simulink model "LinearizedQuadModel"  (R2015b)
settings: Solver=ode45  StartTime=0.0  StopTime=400  RelTol=1e-3
values from neighbouring files (symbols this model uses):
  b_ = 3.13E-5    (= 3.13e-05)    [LinearizedQuad.m]
  Iyy = 6.228E-3    (= 0.006228)    [LinearizedQuad.m]
  Klqr_i = lqr(A_aug,B_aug, Q2, R)    [LinearizedQuad.m]
  Klqr_i_2 = lqr(A_aug2,B_aug2, Q_2i, R_2)    [LinearizedQuad.m]
  Klqr_x = lqr(Ax, Bx, Qx, Rx)    [LinearizedQuad.m]
  l = 0.232    [LinearizedQuad.m]
  m = 0.53    [LinearizedQuad.m]
undefined symbols (not defined in the file or in its folder): deg, rad, s
libraries: aerolibconvert2 x7, simulink x1
settings Model: Creator=aa13417  LastModifiedBy=Salua
settings DataIOCC: SaveFormat=Array
settings DebuggingCC: UnderspecifiedInitializationDetection=Classic  MergeDetectMultiDrivingBlocksExec=none  SolverPrmCheckMsg=warning  StateNameClashWarn=warning
settings HardwareCC: ProdBitPerPointer=32  ProdLargestAtomicFloat=None  ProdIntDivRoundTo=Undefined  ProdEndianess=Unspecified  ProdWordSize=32  ProdHWDeviceType=32-bit Generic
settings GRTTargetCC: GeneratePreprocessorConditionals=Disable all
settings ConfigComp: CovModelRefEnable=Off

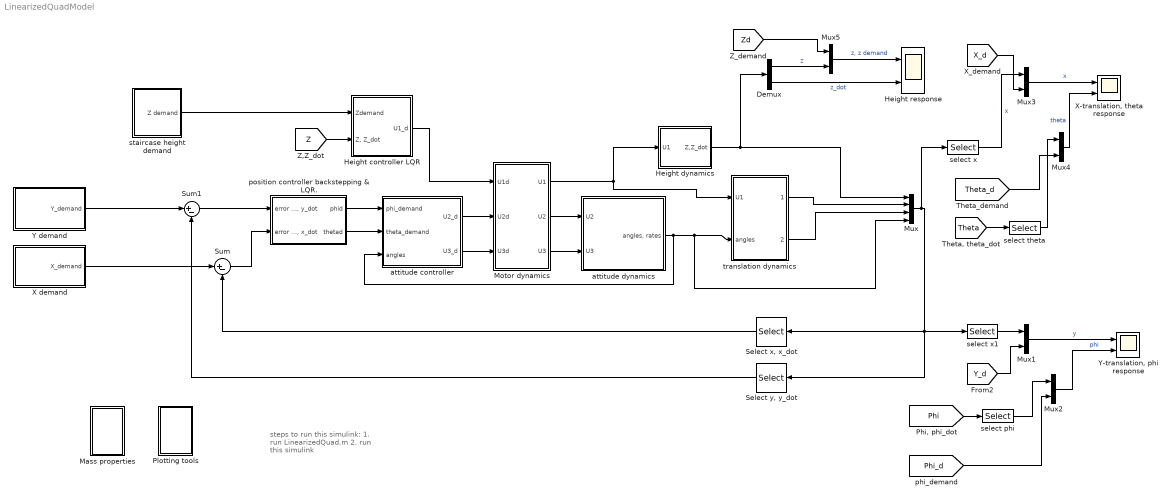
== system LinearizedQuadModel ==
  note: steps to run this simulink:
      | 1. run LinearizedQuad.m
      | 2. run this simulink
  Demux : Demux  Outputs=2
  Height controller LQR : Subsystem
  Height dynamics : Subsystem
  Height response : Scope  NumInputPorts=2
  Mass properties : Subsystem
  Motor dynamics : Subsystem
  Mux : Mux
  Mux{1..5} (5 alike) : Mux  Inputs=2
  Plotting tools : Subsystem
  "Select x, x_dot" : Selector  InputPortWidth=10  IndexOptions=Index vector (dialog)  Indices=[3, 4]  OutputSizes=1
  "Select y, y_dot" : Selector  InputPortWidth=10  IndexOptions=Index vector (dialog)  Indices=[5, 6]  OutputSizes=1
  Sum : Sum  Inputs=|+-
  Sum1 : Sum  Inputs=|+-
  "X demand " : Subsystem
  "X-translation, theta response" : Scope  NumInputPorts=2
  "Y demand " : Subsystem
  "Y-translation, phi response" : Scope  NumInputPorts=2
  attitude controller : Subsystem
  attitude dynamics : Subsystem
  position controller backstepping & LQR. : Subsystem
  select phi : Selector  InputPortWidth=2  IndexOptions=Index vector (dialog)  Indices=1  OutputSizes=1
  select theta : Selector  InputPortWidth=2  IndexOptions=Index vector (dialog)  Indices=1  OutputSizes=1
  select x : Selector  InputPortWidth=10  IndexOptions=Index vector (dialog)  Indices=3  OutputSizes=1
  select x1 : Selector  InputPortWidth=10  IndexOptions=Index vector (dialog)  Indices=5  OutputSizes=1
  staircase height demand : Subsystem
  translation dynamics : Subsystem
  wires:
  Height dynamics/1(Z,Z_dot) -> Mux/1, Demux/1
  attitude dynamics/1("angles, rates") -> attitude controller/3(angles), Mux/4, translation dynamics/2(angles)
  translation dynamics/1("X, X_dot") -> Mux/2
  Mux/1 -> select x/1, select x1/1, "Select x, x_dot"/1, "Select y, y_dot"/1
  "Select x, x_dot"/1 -> Sum/2
  Height controller LQR/1(U1_d) -> Motor dynamics/1(U1d)
  attitude controller/2(U3_d) -> Motor dynamics/3(U3d)
  Motor dynamics/1(U1) -> translation dynamics/1(U1), Height dynamics/1(U1)
  Demux/2 -> Height response/2  "z_dot"
  [Z] -> Height controller LQR/2("Z, Z_dot")
  Motor dynamics/3(U3) -> attitude dynamics/2(U3)
  translation dynamics/2("Y, Y_dot") -> Mux/3
  "Select y, y_dot"/1 -> Sum1/2
  attitude controller/1(U2_d) -> Motor dynamics/2(U2d)
  Motor dynamics/2(U2) -> attitude dynamics/1("U2 ")
  staircase height demand/1(Z demand) -> Height controller LQR/1(Zdemand)
  select x/1 -> Mux3/1  "x"
  [X_d] -> Mux3/2
  Mux3/1 -> "X-translation, theta response"/1  "x"
  [Theta_d] -> Mux4/2
  Mux4/1 -> "X-translation, theta response"/2  "theta"
  [Theta] -> select theta/1
  select theta/1 -> Mux4/1
  position controller backstepping & LQR./2(thetad) -> attitude controller/2(theta_demand)
  position controller backstepping & LQR./1(phid) -> attitude controller/1(phi_demand)
  select x1/1 -> Mux1/1
  [Y_d] -> Mux1/2
  Mux1/1 -> "Y-translation, phi response"/1  "y"
  Mux2/1 -> "Y-translation, phi response"/2  "phi"
  [Phi] -> select phi/1
  select phi/1 -> Mux2/1
  [Phi_d] -> Mux2/2
  [Zd] -> Mux5/1
  Demux/1 -> Mux5/2  "z"
  Mux5/1 -> Height response/1  "z, z demand"
  "Y demand "/1(Y_demand) -> Sum1/1
  "X demand "/1(X_demand) -> Sum/1
  Sum1/1 -> position controller backstepping & LQR./1("error y, y_dot")
  Sum/1 -> position controller backstepping & LQR./2("error x, x_dot")

== system LinearizedQuadModel/Height controller LQR ==
  Zdemand : Inport
  "Z, Z_dot" : Inport  Port=2
  LQR control : Subsystem
  U1_d : Outport
  wires:
  Zdemand/1 -> LQR control/1(Zd)
  LQR control/1(U1d) -> U1_d/1
  "Z, Z_dot"/1 -> LQR control/2(states)

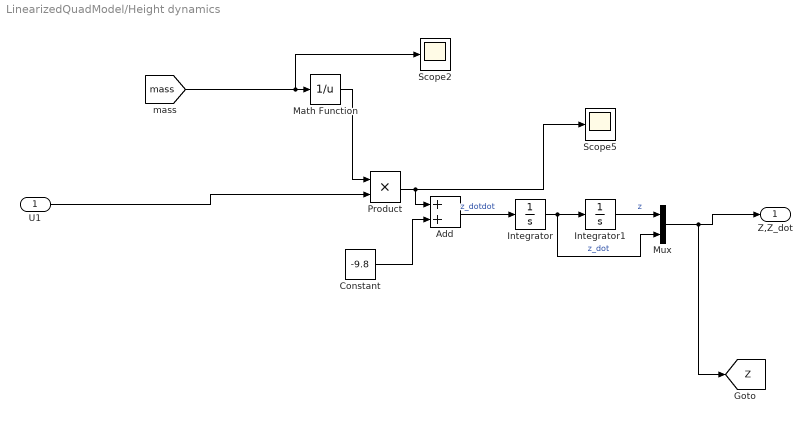
== system LinearizedQuadModel/Height dynamics ==
  U1 : Inport
  Add : Sum
  Constant : Constant  Value=-9.8
  Integrator : Integrator
  Integrator1 : Integrator
  Math Function : Math  Operator=reciprocal  SaturateOnIntegerOverflow=on
  Mux : Mux  Inputs=2
  Product : Product
  Scope2 : Scope
  Scope5 : Scope
  Z,Z_dot : Outport
  tag scope: Z=global
  wires:
  Integrator/1 -> Mux/2, Integrator1/1  "z_dot"
  Product/1 -> Scope5/1, Add/1
  [mass] -> Scope2/1, Math Function/1
  Math Function/1 -> Product/1
  Integrator1/1 -> Mux/1  "z"
  Mux/1 -> [Z], Z,Z_dot/1
  Add/1 -> Integrator/1  "z_dotdot"
  Constant/1 -> Add/2
  U1/1 -> Product/2

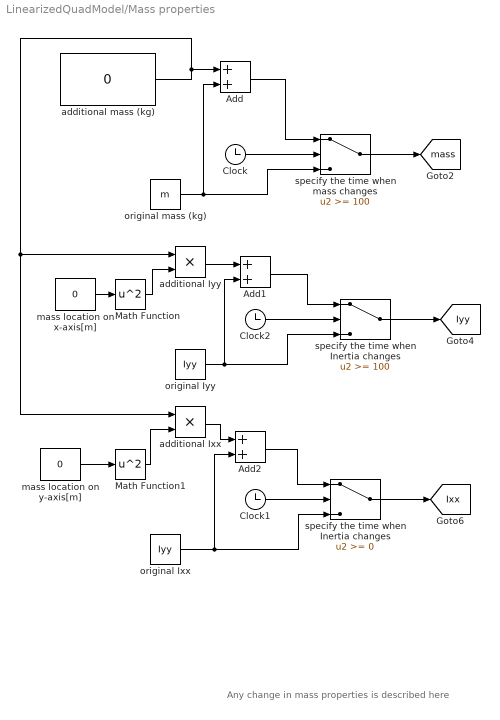
== system LinearizedQuadModel/Mass properties ==
  note: Any change in mass properties is described here
  Add : Sum
  Add1 : Sum
  Add2 : Sum
  Clock : Clock
  Clock1 : Clock
  Clock2 : Clock
  Math Function : Math  Operator=square  SaturateOnIntegerOverflow=on
  Math Function1 : Math  Operator=square  SaturateOnIntegerOverflow=on
  additional Ixx : Product  Inputs=**
  additional Iyy : Product  Inputs=**
  additional mass (kg) : Constant  Value=0
  mass location on x-axis[m] : Constant  Value=0
  mass location on y-axis[m] : Constant  Value=0
  original Ixx : Constant  Value=Iyy
  original Iyy : Constant  Value=Iyy
  original mass (kg) : Constant  Value=m
  specify the time when Inertia changes : Switch  Threshold=100
  "specify the time when Inertia changes  " : Switch
  specify the time when mass changes : Switch  Threshold=100
  tag scope: Ixx=global, Iyy=global, mass=global
  wires:
  Add/1 -> specify the time when mass changes/1
  specify the time when mass changes/1 -> [mass]
  original mass (kg)/1 -> specify the time when mass changes/3, Add/2
  Clock/1 -> specify the time when mass changes/2
  Add1/1 -> specify the time when Inertia changes/1
  specify the time when Inertia changes/1 -> [Iyy]
  original Iyy/1 -> Add1/2, specify the time when Inertia changes/3
  Clock2/1 -> specify the time when Inertia changes/2
  additional mass (kg)/1 -> additional Iyy/1, additional Ixx/1, Add/1
  mass location on x-axis[m]/1 -> Math Function/1
  additional Iyy/1 -> Add1/1
  "specify the time when Inertia changes  "/1 -> [Ixx]
  Clock1/1 -> "specify the time when Inertia changes  "/2
  original Ixx/1 -> Add2/2, "specify the time when Inertia changes  "/3
  Add2/1 -> "specify the time when Inertia changes  "/1
  mass location on y-axis[m]/1 -> Math Function1/1
  additional Ixx/1 -> Add2/1
  Math Function/1 -> additional Iyy/2
  Math Function1/1 -> additional Ixx/2

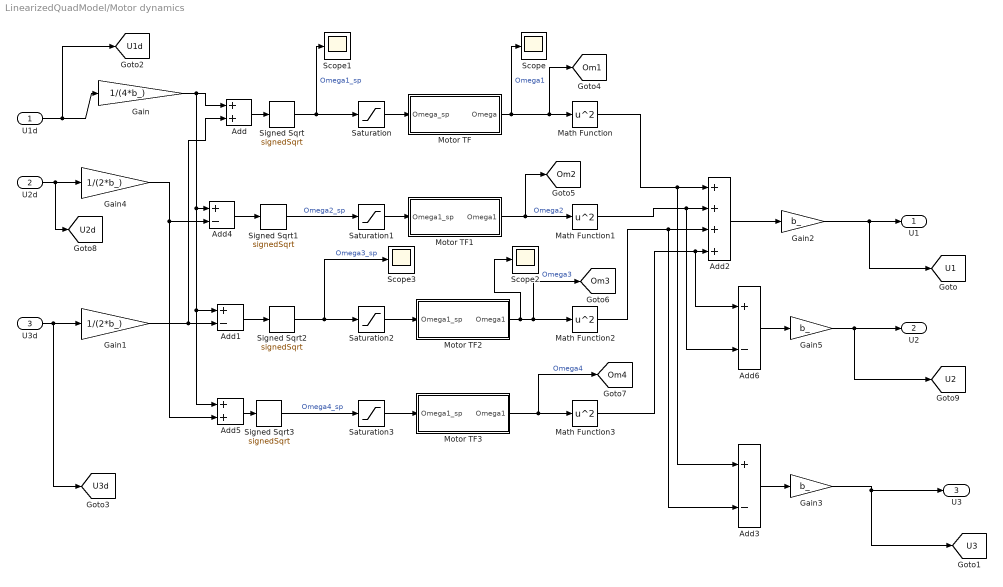
== system LinearizedQuadModel/Motor dynamics ==
  U1d : Inport
  U2d : Inport  Port=2
  U3d : Inport  Port=3
  Add : Sum
  Add{1,3..4,6} (4 alike) : Sum  Inputs=+-
  Add2 : Sum  Inputs=++++
  Add5 : Sum
  Gain : Gain  Gain=1/(4*b_)
  Gain1 : Gain  Gain=1/(2*b_)
  Gain2 : Gain  Gain=b_
  Gain3 : Gain  Gain=b_
  Gain4 : Gain  Gain=1/(2*b_)
  Gain5 : Gain  Gain=b_
  Math Function{,1..3} (4 alike) : Math  Operator=square  SaturateOnIntegerOverflow=on
  Motor TF : Subsystem
  Motor TF1 : Subsystem
  Motor TF2 : Subsystem
  Motor TF3 : Subsystem
  Saturation{,1..3} (4 alike) : Saturate  UpperLimit=341  LowerLimit=24
  Scope{,1..3} (4 alike) : Scope
  Signed Sqrt{,1..3} (4 alike) : Sqrt  Operator=signedSqrt  OutputSignalType=real  SaturateOnIntegerOverflow=on
  U1 : Outport
  U2 : Outport  Port=2
  U3 : Outport  Port=3
  tag scope: Om1=global, Om2=global, Om3=global, Om4=global, U1=global, U1d=global, U2=global, U2d=global, U3=global, U3d=global
  wires:
  U3d/1 -> [U3d], Gain1/1
  Motor TF/1(Omega) -> Scope/1, [Om1], Math Function/1  "Omega1"
  Saturation/1 -> Motor TF/1(Omega_sp)
  Gain/1 -> Add5/1, Add1/1, Add4/1, Add/1
  U1d/1 -> [U1d], Gain/1
  Add/1 -> Signed Sqrt/1
  Math Function/1 -> Add2/1, Add3/1
  Signed Sqrt/1 -> Scope1/1, Saturation/1  "Omega1_sp"
  Gain1/1 -> Add/2, Add1/2
  Signed Sqrt1/1 -> Saturation1/1  "Omega2_sp"
  Saturation1/1 -> Motor TF1/1(Omega1_sp)
  Add1/1 -> Signed Sqrt2/1
  Signed Sqrt2/1 -> Scope3/1, Saturation2/1  "Omega3_sp"
  Saturation2/1 -> Motor TF2/1(Omega1_sp)
  Motor TF2/1(Omega1) -> Scope2/1, [Om3], Math Function2/1  "Omega3"
  Signed Sqrt3/1 -> Saturation3/1  "Omega4_sp"
  Saturation3/1 -> Motor TF3/1(Omega1_sp)
  Motor TF3/1(Omega1) -> [Om4], Math Function3/1  "Omega4"
  Math Function3/1 -> Add6/1, Add2/4
  Math Function2/1 -> Add3/2, Add2/3
  Math Function1/1 -> Add2/2, Add6/2
  Add2/1 -> Gain2/1
  Gain2/1 -> [U1], U1/1
  Add3/1 -> Gain3/1
  Gain3/1 -> U3/1, [U3]
  Motor TF1/1(Omega1) -> [Om2], Math Function1/1  "Omega2"
  U2d/1 -> Gain4/1, [U2d]
  Gain4/1 -> Add5/2, Add4/2
  Add4/1 -> Signed Sqrt1/1
  Add5/1 -> Signed Sqrt3/1
  Add6/1 -> Gain5/1
  Gain5/1 -> [U2], U2/1

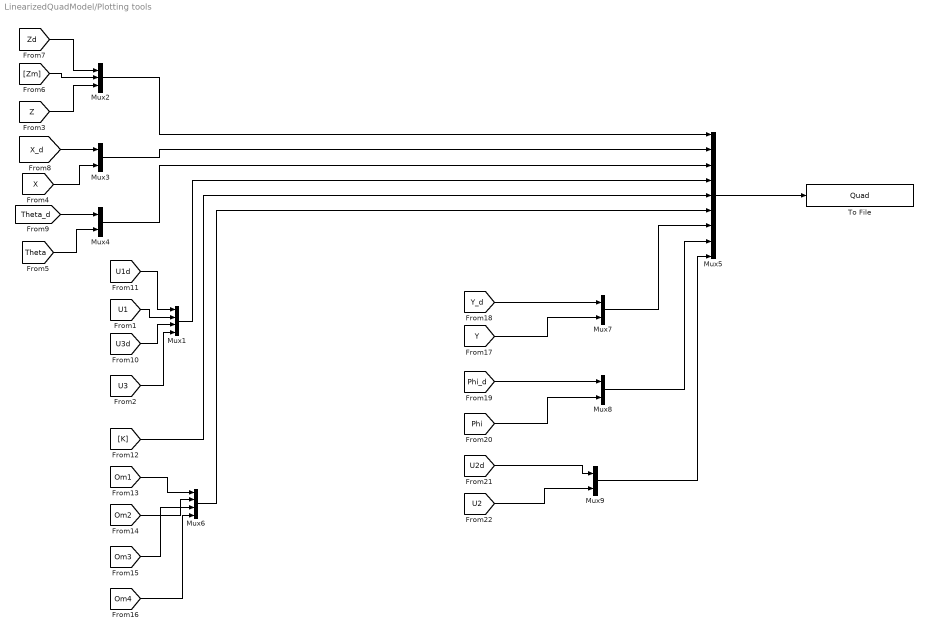
== system LinearizedQuadModel/Plotting tools ==
  Mux1 : Mux
  Mux2 : Mux  Inputs=3
  Mux{3..4,7..9} (5 alike) : Mux  Inputs=2
  Mux5 : Mux  Inputs=9
  Mux6 : Mux
  To File : ToFile  Filename=Quad  MatrixName=simoutput2  SaveFormat=Timeseries
  wires:
  [Om3] -> Mux6/3
  [Z] -> Mux2/3
  Mux3/1 -> Mux5/2
  Mux1/1 -> Mux5/4
  [Zm] -> Mux2/2
  [Zd] -> Mux2/1
  [U3d] -> Mux1/3
  [U3] -> Mux1/4
  Mux5/1 -> To File/1
  [Om2] -> Mux6/2
  [Om4] -> Mux6/4
  [X_d] -> Mux3/1
  [X] -> Mux3/2
  [U1d] -> Mux1/1
  Mux6/1 -> Mux5/6
  Mux2/1 -> Mux5/1
  [Om1] -> Mux6/1
  [U1] -> Mux1/2
  [Theta_d] -> Mux4/1
  Mux4/1 -> Mux5/3
  [K] -> Mux5/5
  [Theta] -> Mux4/2
  [Y_d] -> Mux7/1
  [Y] -> Mux7/2
  [Phi_d] -> Mux8/1
  [Phi] -> Mux8/2
  [U2d] -> Mux9/1
  [U2] -> Mux9/2
  Mux7/1 -> Mux5/7
  Mux8/1 -> Mux5/8
  Mux9/1 -> Mux5/9

== system LinearizedQuadModel/X demand  ==
  Mux1 : Mux  Inputs=2
  demand start time : Subsystem
  x_demand : Constant  Value=0
  x_dot demand (default 0) : Constant  Value=0
  X_demand : Outport
  tag scope: X_d=global
  wires:
  x_demand/1 -> Mux1/1, [X_d]
  Mux1/1 -> demand start time/1(In1)
  x_dot demand (default 0)/1 -> Mux1/2
  demand start time/1(Out1) -> X_demand/1

== system LinearizedQuadModel/Y demand  ==
  Mux2 : Mux  Inputs=2
  demand start time : Subsystem
  y_demand : Constant  Value=0
  y_dot demand (default 0) : Constant  Value=0
  Y_demand : Outport
  tag scope: Y_d=global
  wires:
  Mux2/1 -> demand start time/1(In1)
  y_demand/1 -> [Y_d], Mux2/1
  y_dot demand (default 0)/1 -> Mux2/2
  demand start time/1(Out1) -> Y_demand/1

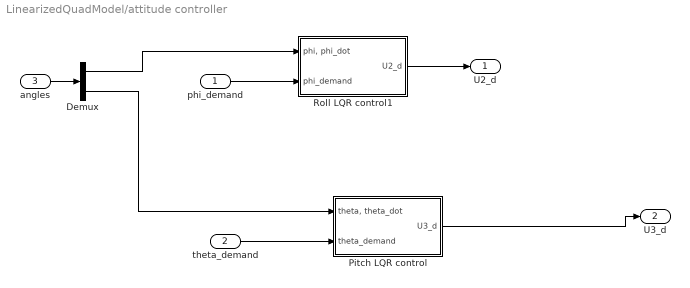
== system LinearizedQuadModel/attitude controller ==
  phi_demand : Inport
  theta_demand : Inport  Port=2
  angles : Inport  Port=3
  Demux : Demux  Outputs=[2,2]
  Pitch LQR control : Subsystem
  Roll LQR control1 : Subsystem
  U2_d : Outport
  U3_d : Outport  Port=2
  wires:
  theta_demand/1 -> Pitch LQR control/2(theta_demand)
  Roll LQR control1/1(U2_d) -> U2_d/1
  phi_demand/1 -> Roll LQR control1/2(phi_demand)
  angles/1 -> Demux/1
  Demux/1 -> Roll LQR control1/1("phi, phi_dot")
  Demux/2 -> Pitch LQR control/1("theta, theta_dot")
  Pitch LQR control/1(U3_d) -> U3_d/1

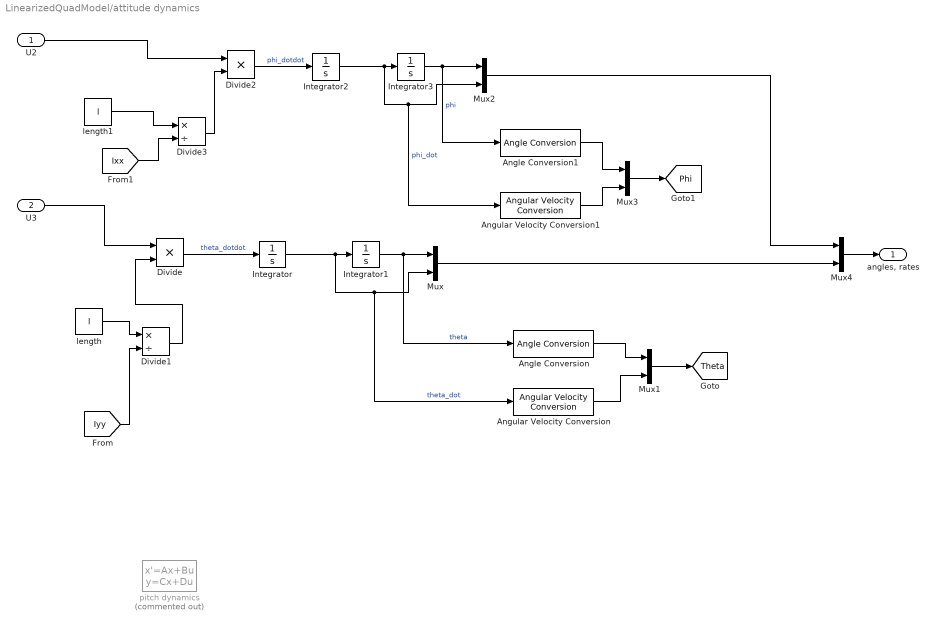
== system LinearizedQuadModel/attitude dynamics ==
  "U2 " : Inport
  U3 : Inport  Port=2
  Angle Conversion : aerolibconvert2/Angle Conversion  IU=rad  OU=deg
  Angle Conversion1 : aerolibconvert2/Angle Conversion  IU=rad  OU=deg
  Angular Velocity Conversion : aerolibconvert2/Angular Velocity Conversion  IU=rad/s  OU=deg/s
  Angular Velocity Conversion1 : aerolibconvert2/Angular Velocity Conversion  IU=rad/s  OU=deg/s
  Divide : Product  Inputs=**
  Divide1 : Product  Inputs=*/
  Divide2 : Product  Inputs=**
  Divide3 : Product  Inputs=*/
  Integrator{,1..3} (4 alike) : Integrator
  Mux{,1..4} (5 alike) : Mux  Inputs=2
  length : Constant  Value=l
  length1 : Constant  Value=l
  pitch dynamics : StateSpace  Commented=on  A=|  B=|  C=eye(2)  D=zeros(2,1)  X0=0
      A=|
      | [0 1;
      |        0 0]
      B=|
      | [0;
      |        l/Iyy]
  "angles, rates" : Outport
  tag scope: Phi=global, Theta=global
  wires:
  U3/1 -> Divide/1
  length/1 -> Divide1/1
  Divide/1 -> Integrator/1  "theta_dotdot"
  Integrator/1 -> Angular Velocity Conversion/1, Mux/2, Integrator1/1  "theta_dot"
  Integrator1/1 -> Angle Conversion/1, Mux/1  "theta"
  Mux/1 -> Mux4/2
  [Iyy] -> Divide1/2
  Divide1/1 -> Divide/2
  Angle Conversion/1 -> Mux1/1
  Mux1/1 -> [Theta]
  Angular Velocity Conversion/1 -> Mux1/2
  length1/1 -> Divide3/1
  [Ixx] -> Divide3/2
  Divide3/1 -> Divide2/2
  "U2 "/1 -> Divide2/1
  Divide2/1 -> Integrator2/1  "phi_dotdot"
  Integrator2/1 -> Angular Velocity Conversion1/1, Mux2/2, Integrator3/1  "phi_dot"
  Integrator3/1 -> Angle Conversion1/1, Mux2/1  "phi"
  Angle Conversion1/1 -> Mux3/1
  Angular Velocity Conversion1/1 -> Mux3/2
  Mux3/1 -> [Phi]
  Mux2/1 -> Mux4/1
  Mux4/1 -> "angles, rates"/1

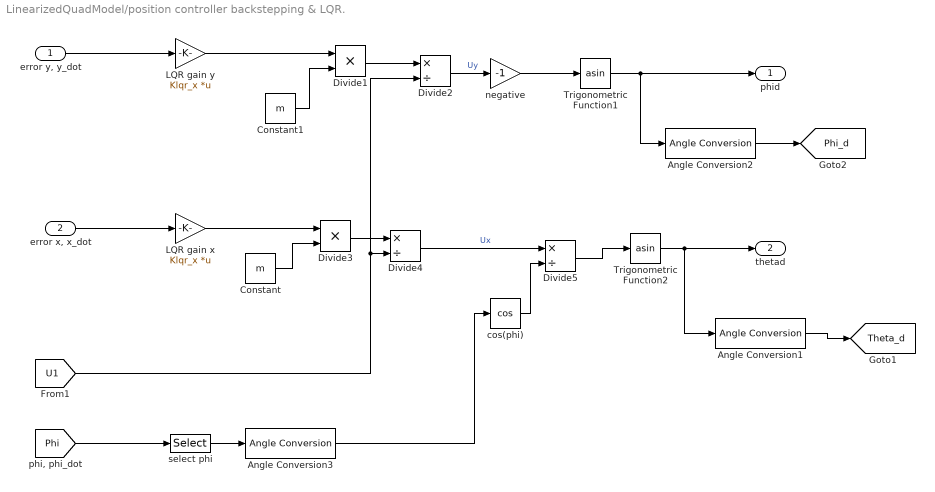
== system LinearizedQuadModel/position controller backstepping & LQR. ==
  "error y, y_dot" : Inport
  "error x, x_dot" : Inport  Port=2
  Angle Conversion1 : aerolibconvert2/Angle Conversion  IU=rad  OU=deg
  Angle Conversion2 : aerolibconvert2/Angle Conversion  IU=rad  OU=deg
  Angle Conversion3 : aerolibconvert2/Angle Conversion  IU=deg  OU=rad
  Constant : Constant  Value=m
  Constant1 : Constant  Value=m
  Divide1 : Product  Inputs=**
  Divide2 : Product  Inputs=*/
  Divide3 : Product  Inputs=**
  Divide4 : Product  Inputs=*/
  Divide5 : Product  Inputs=*/
  LQR gain x : Gain  Gain=Klqr_x  Multiplication=Matrix(K*u)
  LQR gain y : Gain  Gain=Klqr_x  Multiplication=Matrix(K*u)
  Trigonometric Function1 : Trigonometry  Operator=asin
  Trigonometric Function2 : Trigonometry  Operator=asin
  cos(phi) : Trigonometry  Operator=cos
  negative : Gain  Gain=-1
  select phi : Selector  InputPortWidth=2  IndexOptions=Index vector (dialog)  Indices=1  OutputSizes=1
  phid : Outport
  thetad : Outport  Port=2
  tag scope: Phi_d=global, Theta_d=global
  wires:
  Angle Conversion1/1 -> [Theta_d]
  Trigonometric Function2/1 -> thetad/1, Angle Conversion1/1
  Constant/1 -> Divide3/2
  Divide3/1 -> Divide4/1
  [U1] -> Divide2/2, Divide4/2
  Divide4/1 -> Divide5/1  "Ux"
  "error y, y_dot"/1 -> LQR gain y/1
  LQR gain y/1 -> Divide1/1
  Constant1/1 -> Divide1/2
  Divide1/1 -> Divide2/1
  Divide2/1 -> negative/1  "Uy"
  negative/1 -> Trigonometric Function1/1
  Trigonometric Function1/1 -> Angle Conversion2/1, phid/1
  Angle Conversion2/1 -> [Phi_d]
  select phi/1 -> Angle Conversion3/1
  cos(phi)/1 -> Divide5/2
  Divide5/1 -> Trigonometric Function2/1
  LQR gain x/1 -> Divide3/1
  "error x, x_dot"/1 -> LQR gain x/1
  [Phi] -> select phi/1
  Angle Conversion3/1 -> cos(phi)/1

== system LinearizedQuadModel/staircase height demand ==
  Add : Sum
  Rate Transition : RateTransition
  min height demand : Constant
  z demand : simulink/Sources/Repeating Sequence Stair  OutValues=[2 2 2 2 2 2].'  tsamp=20  OutMin=[]  OutMax=[]  OutDataTypeStr=double  OutputDataTypeScalingMode=double  OutDataType=fixdt(0,8)  ConRadixGroup=Best Precision: Vector-wise  OutScaling=2^-12
  Z demand : Outport
  tag scope: Zd=global
  wires:
  Add/1 -> [Zd], Z demand/1
  Rate Transition/1 -> Add/1
  z demand/1 -> Rate Transition/1
  min height demand/1 -> Add/2

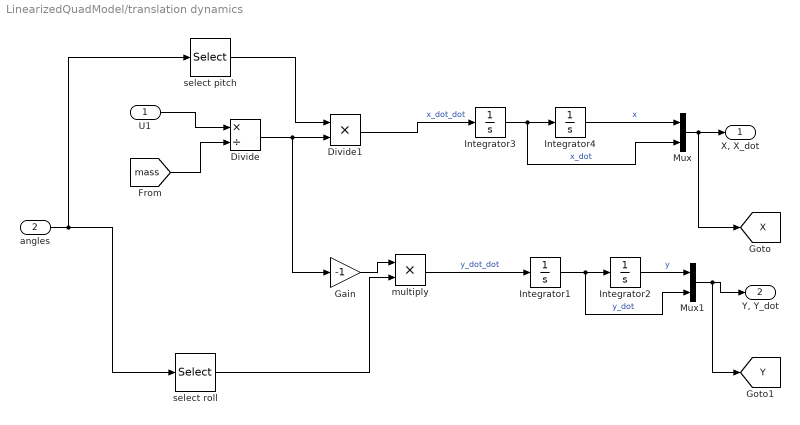
== system LinearizedQuadModel/translation dynamics ==
  U1 : Inport
  angles : Inport  Port=2
  Divide : Product  Inputs=*/
  Divide1 : Product  Inputs=**
  Gain : Gain  Gain=-1
  Integrator{1..4} (4 alike) : Integrator
  Mux : Mux  Inputs=2
  Mux1 : Mux  Inputs=2
  multiply : Product  Inputs=**
  select pitch : Selector  InputPortWidth=4  IndexOptions=Index vector (dialog)  Indices=3  OutputSizes=1
  "select roll " : Selector  InputPortWidth=4  IndexOptions=Index vector (dialog)  Indices=1  OutputSizes=1
  "X, X_dot" : Outport
  "Y, Y_dot" : Outport  Port=2
  tag scope: X=global, Y=global
  wires:
  Integrator3/1 -> Mux/2, Integrator4/1  "x_dot"
  Divide1/1 -> Integrator3/1  "x_dot_dot"
  select pitch/1 -> Divide1/1
  Integrator4/1 -> Mux/1  "x"
  Mux/1 -> [X], "X, X_dot"/1
  [mass] -> Divide/2
  U1/1 -> Divide/1
  Divide/1 -> Gain/1, Divide1/2
  "select roll "/1 -> multiply/2
  Gain/1 -> multiply/1
  multiply/1 -> Integrator1/1  "y_dot_dot"
  Integrator1/1 -> Mux1/2, Integrator2/1  "y_dot"
  Integrator2/1 -> Mux1/1  "y"
  Mux1/1 -> [Y], "Y, Y_dot"/1
  angles/1 -> select pitch/1, "select roll "/1

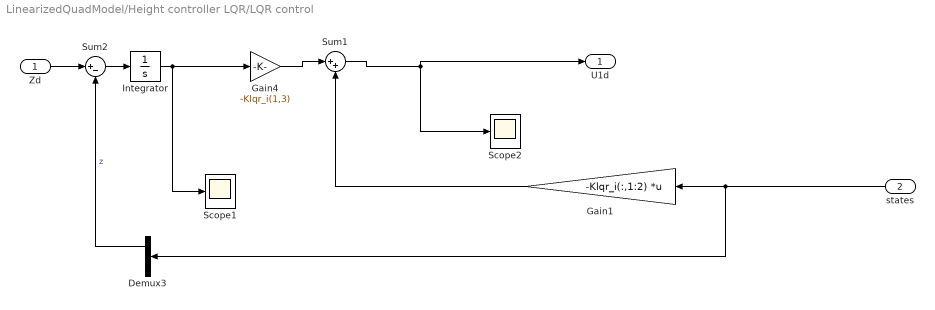
== system LinearizedQuadModel/Height controller LQR/LQR control ==
  Zd : Inport
  states : Inport  Port=2
  Demux3 : Demux  Outputs=[1,1]
  Gain1 : Gain  Gain=-Klqr_i(:,1:2)  Multiplication=Matrix(K*u)
  Gain4 : Gain  Gain=-Klqr_i(1,3)
  Integrator : Integrator  InitialCondition=6
  Scope1 : Scope
  Scope2 : Scope
  Sum1 : Sum  Inputs=|++
  Sum2 : Sum  Inputs=|+-
  U1d : Outport
  wires:
  Zd/1 -> Sum2/1
  Gain1/1 -> Sum1/2
  Integrator/1 -> Scope1/1, Gain4/1
  Gain4/1 -> Sum1/1
  states/1 -> Demux3/1, Gain1/1
  Sum1/1 -> U1d/1, Scope2/1
  Demux3/1 -> Sum2/2  "z"
  Sum2/1 -> Integrator/1

== system LinearizedQuadModel/Motor dynamics/Motor TF ==
  Omega_sp : Inport
  Gain2 : Gain  Gain=1.0683
  Gain3 : Gain  Gain=5.2584
  Integrator : Integrator  InitialCondition=203.68  LimitOutput=on
  Sum1 : Sum  Inputs=|+-
  Omega : Outport
  wires:
  Integrator/1 -> Omega/1, Gain2/1
  Gain2/1 -> Sum1/2
  Gain3/1 -> Integrator/1
  Sum1/1 -> Gain3/1
  Omega_sp/1 -> Sum1/1

== system LinearizedQuadModel/Motor dynamics/Motor TF1 ==
  Omega1_sp : Inport
  Gain2 : Gain  Gain=1.0683
  Gain3 : Gain  Gain=5.2584
  Integrator : Integrator  InitialCondition=203.68  LimitOutput=on
  Sum1 : Sum  Inputs=|+-
  Omega1 : Outport
  wires:
  Omega1_sp/1 -> Sum1/1
  Sum1/1 -> Gain3/1
  Gain3/1 -> Integrator/1
  Gain2/1 -> Sum1/2
  Integrator/1 -> Gain2/1, Omega1/1

== system LinearizedQuadModel/Motor dynamics/Motor TF2 ==
  Omega1_sp : Inport
  Gain2 : Gain  Gain=1.0683
  Gain3 : Gain  Gain=5.2584
  Integrator : Integrator  InitialCondition=203.68  LimitOutput=on
  Sum1 : Sum  Inputs=|+-
  Omega1 : Outport
  wires:
  Integrator/1 -> Omega1/1, Gain2/1
  Gain2/1 -> Sum1/2
  Gain3/1 -> Integrator/1
  Sum1/1 -> Gain3/1
  Omega1_sp/1 -> Sum1/1

== system LinearizedQuadModel/Motor dynamics/Motor TF3 ==
  Omega1_sp : Inport
  Gain2 : Gain  Gain=1.0683
  Gain3 : Gain  Gain=5.2584
  Integrator : Integrator  InitialCondition=203.68  LimitOutput=on
  Sum1 : Sum  Inputs=|+-
  Omega1 : Outport
  wires:
  Omega1_sp/1 -> Sum1/1
  Sum1/1 -> Gain3/1
  Gain3/1 -> Integrator/1
  Gain2/1 -> Sum1/2
  Integrator/1 -> Gain2/1, Omega1/1

== system LinearizedQuadModel/X demand /demand start time ==
  In1 : Inport
  Clock1 : Clock
  Switch : Switch  Threshold=59
  x_dot demand1 : Constant  Value=0
  Out1 : Outport
  wires:
  Clock1/1 -> Switch/2
  x_dot demand1/1 -> Switch/3
  Switch/1 -> Out1/1
  In1/1 -> Switch/1

== system LinearizedQuadModel/Y demand /demand start time ==
  In1 : Inport
  Clock1 : Clock
  Switch : Switch  Threshold=20
  x_dot demand1 : Constant  Value=0
  Out1 : Outport
  wires:
  In1/1 -> Switch/1
  Switch/1 -> Out1/1
  x_dot demand1/1 -> Switch/3
  Clock1/1 -> Switch/2

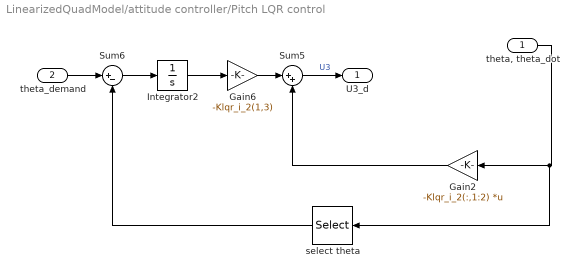
== system LinearizedQuadModel/attitude controller/Pitch LQR control ==
  "theta, theta_dot" : Inport
  theta_demand : Inport  Port=2
  Gain2 : Gain  Gain=-Klqr_i_2(:,1:2)  Multiplication=Matrix(K*u)
  Gain6 : Gain  Gain=-Klqr_i_2(1,3)
  Integrator2 : Integrator
  Sum5 : Sum  Inputs=|++
  Sum6 : Sum  Inputs=|+-
  select theta : Selector  InputPortWidth=2  IndexOptions=Index vector (dialog)  Indices=1  OutputSizes=1
  U3_d : Outport
  wires:
  Sum5/1 -> U3_d/1  "U3"
  Gain2/1 -> Sum5/2
  Gain6/1 -> Sum5/1
  select theta/1 -> Sum6/2
  Sum6/1 -> Integrator2/1
  Integrator2/1 -> Gain6/1
  theta_demand/1 -> Sum6/1
  "theta, theta_dot"/1 -> Gain2/1, select theta/1

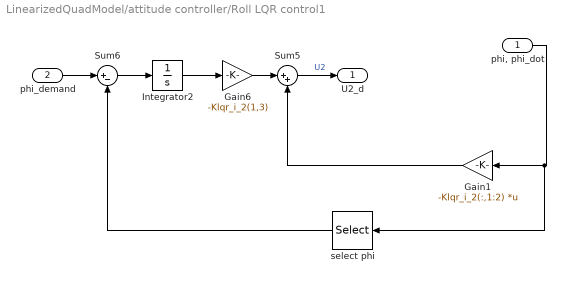
== system LinearizedQuadModel/attitude controller/Roll LQR control1 ==
  "phi, phi_dot" : Inport
  phi_demand : Inport  Port=2
  Gain1 : Gain  Gain=-Klqr_i_2(:,1:2)  Multiplication=Matrix(K*u)
  Gain6 : Gain  Gain=-Klqr_i_2(1,3)
  Integrator2 : Integrator
  Sum5 : Sum  Inputs=|++
  Sum6 : Sum  Inputs=|+-
  select phi : Selector  InputPortWidth=2  IndexOptions=Index vector (dialog)  Indices=1  OutputSizes=1
  U2_d : Outport
  wires:
  "phi, phi_dot"/1 -> Gain1/1, select phi/1
  phi_demand/1 -> Sum6/1
  Integrator2/1 -> Gain6/1
  Sum6/1 -> Integrator2/1
  select phi/1 -> Sum6/2
  Gain6/1 -> Sum5/1
  Gain1/1 -> Sum5/2
  Sum5/1 -> U2_d/1  "U2"
